simulink model "e1p3b"  (R2017a)
settings: Solver=VariableStepAuto  StartTime=0.0  StopTime=10.0  RelTol=1e-3
values from neighbouring files (symbols this model uses):
  A = [-0.0000 1.0000 -0.0000 0.0000 ... (first row only)    [e1p3.m]    (also in e1p3a.m)
  B = [-0.0000 -0.0000 ... (first row only)    [e1p3.m]    (also in e1p3a.m)
  C = eye(4)    [e1p3.m]    (also in e1p3a.m)
  D = zeros(4,2)    [e1p3.m]    (also in e1p3a.m)
undefined symbols (not defined in the file or in its folder): K
settings Model: Creator=Soutrik  LastModifiedBy=Soutrik

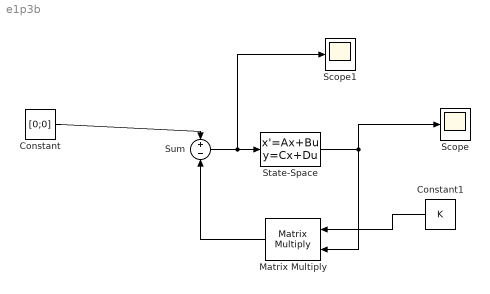
== system e1p3b ==
  Constant : Constant  Value=[0;0]
  Constant1 : Constant  Value=K
  Matrix Multiply : Product  Multiplication=Matrix(*)
  Scope : Scope
  Scope1 : Scope
  State-Space : StateSpace  A=A  B=B  C=C  D=D  X0=[0.01 0 0 0]
  Sum : Sum  Inputs=+-
  wires:
  State-Space/1 -> Matrix Multiply/2, Scope/1
  Constant/1 -> Sum/1
  Sum/1 -> Scope1/1, State-Space/1
  Matrix Multiply/1 -> Sum/2
  Constant1/1 -> Matrix Multiply/1
